simulink model "vor_block_diagram"  (Simulink 8.8)
settings: Solver=ode45  StartTime=0.0  StopTime=10.0  RelTol=1e-3  EnableMultiTasking=on
values from neighbouring files (symbols this model uses):
  g = 1    [canal_afferent_step_response.m]
  T = 0.015    [canal_afferent_step_response.m]
  T2 = 0.003    [canal_afferent_step_response.m]
  Ts = simoutTP    [canal_afferent_step_response.m]
undefined symbols (not defined in the file or in its folder): delay, Tc, Te1, Te2, Tvor
settings Model: Creator=hallyment  LastModifiedBy=hallyment
settings OptimizationCC: InitFltsAndDblsToZero=on
settings DebuggingCC: SaveWithParameterizedLinksMsg=none  SignalResolutionControl=TryResolveAllWithWarning  SolverPrmCheckMsg=warning  MultiTaskDSMMsg=warning  MultiTaskCondExecSysMsg=none  StateNameClashWarn=none  StrictBusMsg=None
settings GRTTargetCC: TargetFcnLib=ansi_tfl_tmw.mat  GeneratePreprocessorConditionals=Use local settings

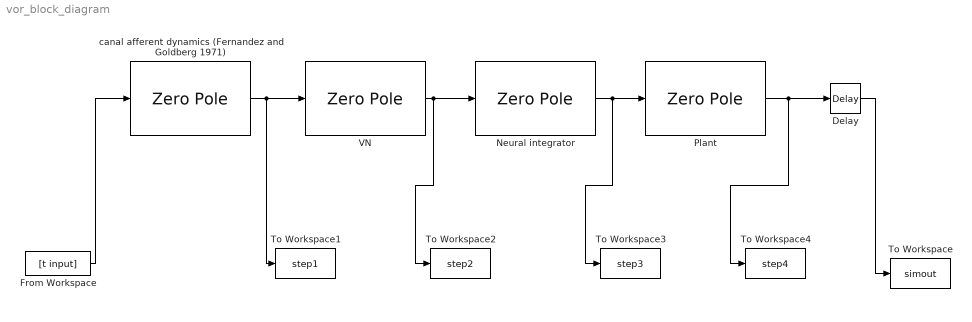
== system vor_block_diagram ==
  Delay : TransportDelay  DelayTime=delay
  From Workspace : FromWorkspace  VariableName=[t input]  SampleTime=Ts
  Neural integrator : ZeroPole  Zeros=[-1/Te1]  Poles=[0]  Gain=[Te1]
  Plant : ZeroPole  Zeros=[0]  Poles=[-1/Te1 -1/Te2]  Gain=[1/(Te1*Te2)]
  To Workspace : ToWorkspace  VariableName=simout  SampleTime=Ts
  To Workspace1 : ToWorkspace  VariableName=step1  SampleTime=Ts
  To Workspace2 : ToWorkspace  VariableName=step2  SampleTime=Ts
  To Workspace3 : ToWorkspace  VariableName=step3  SampleTime=Ts
  To Workspace4 : ToWorkspace  VariableName=step4  SampleTime=Ts
  VN : ZeroPole  Zeros=[-1/Tc]  Poles=[-1/Tvor ]  Gain=[-g]
  canal afferent dynamics (Fernandez and Goldberg 1971) : ZeroPole  Zeros=[ 0 -1/T]  Poles=[-1/Tc -1/T2]  Gain=[T/(Tc*T2)]
  wires:
  Plant/1 -> To Workspace4/1, Delay/1
  Delay/1 -> To Workspace/1
  Neural integrator/1 -> To Workspace3/1, Plant/1
  From Workspace/1 -> canal afferent dynamics (Fernandez and Goldberg 1971)/1
  canal afferent dynamics (Fernandez and Goldberg 1971)/1 -> To Workspace1/1, VN/1
  VN/1 -> To Workspace2/1, Neural integrator/1
